simulink subsystem "xxI_mode"  (R2022a)
settings: Solver=VariableStepAuto  StartTime=0.0  StopTime=10.0  RelTol=1e-3
settings Model: Creator=bkfre  LastModifiedBy=bkfre

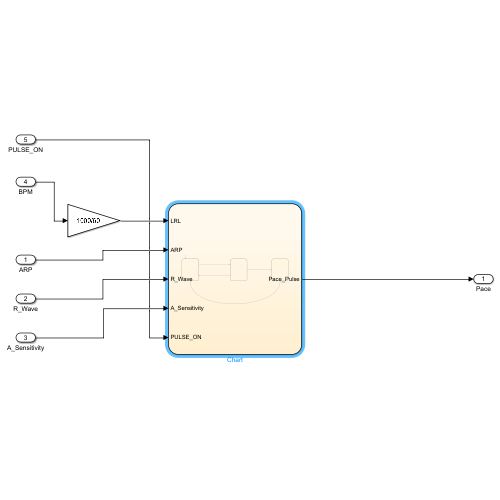
[thumbnail: Simulink's stored preview of the top-level diagram]
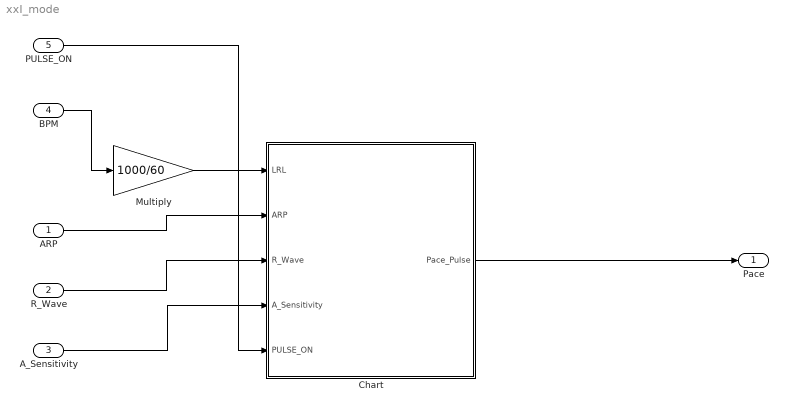
== system xxI_mode ==
  ARP : Inport
  R_Wave : Inport  Port=2
  A_Sensitivity : Inport  Port=3
  BPM : Inport  Port=4
  PULSE_ON : Inport  Port=5
  Chart : Stateflow chart  TreatAsAtomicUnit=on
  Multiply : Gain  Gain=1000/60
  Pace : Outport
  wires:
  R_Wave/1 -> Chart/3(R_Wave)
  Chart/1(Pace_Pulse) -> Pace/1
  A_Sensitivity/1 -> Chart/4(A_Sensitivity)
  ARP/1 -> Chart/2(ARP)
  BPM/1 -> Multiply/1
  Multiply/1 -> Chart/1(LRL)
  PULSE_ON/1 -> Chart/5(PULSE_ON)

== stateflow chart xxI_mode/Chart ==
  state Refractory
    entry:
    Pace_Pulse=0;
  state Alert
  state Pace
    entry:
    Pace_Pulse=1;
  (default) -> Refractory
  Refractory -> Alert : after(ARP-PULSE_ON,msec)
  Alert -> Pace [order 2] : after(LRL-ARP,msec)
  Alert -> Refractory [order 1] : [R_Wave>A_Sensitivity]
  Pace -> Refractory : after(PULSE_ON,msec)
  data: LRL input; ARP input; R_Wave input; Pace_Pulse output; A_Sensitivity input; PULSE_ON input
